simulink model "BlockDiagram3D"  (R2018a)
settings: Solver=VariableStepAuto  StartTime=0.0  StopTime=10.0  RelTol=1e-3
settings Model: Creator=abl010  LastModifiedBy=abl010

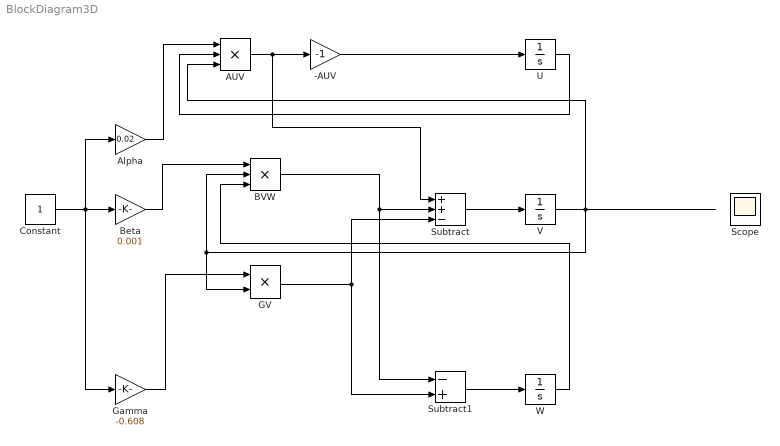
== system BlockDiagram3D ==
  "-AUV " : Gain  Gain=-1
  AUV : Product  Inputs=3
  Alpha : Gain  Gain=0.02
  BVW : Product  Inputs=3
  Beta : Gain  Gain=0.001
  "Constant " : Constant
  GV : Product
  Gamma : Gain  Gain=-0.608
  Scope : Scope
  Subtract : Sum  Inputs=++-
  Subtract1 : Sum  Inputs=-+
  U : Integrator  InitialCondition=100
  V : Integrator  InitialCondition=1
  W : Integrator
  wires:
  "Constant "/1 -> Gamma/1, Beta/1, Alpha/1
  Alpha/1 -> AUV/1
  AUV/1 -> "-AUV "/1, Subtract/1
  U/1 -> AUV/2
  "-AUV "/1 -> U/1
  Subtract/1 -> V/1
  Beta/1 -> BVW/1
  W/1 -> BVW/3
  V/1 -> GV/2, BVW/2, AUV/3
  BVW/1 -> Subtract/2, Subtract1/1
  Gamma/1 -> GV/1
  GV/1 -> Subtract1/2, Subtract/3
  Subtract1/1 -> W/1
